simulink model "Taller4_TDCM"  (R2024a)
settings: Solver=VariableStepAuto  StartTime=0.0  StopTime=0.030  RelTol=1e-3
values from neighbouring files (symbols this model uses):
  A = [0 1; -1/(L*Cap) -R/L]    [Taller4_TCDM.m]    (also in Taller4_TCDM_v2.m)
  B = [0; 1/L]    [Taller4_TCDM.m]    (also in Taller4_TCDM_v2.m)
  C = [1/Cap 0]    [Taller4_TCDM.m]    (also in Taller4_TCDM_v2.m)
  D = 0    [Taller4_TCDM.m]    (also in Taller4_TCDM_v2.m)
  x0 = [0; 0]    [Taller4_TCDM_v2.m]
settings Model: Creator=emili  LastModifiedBy=emili

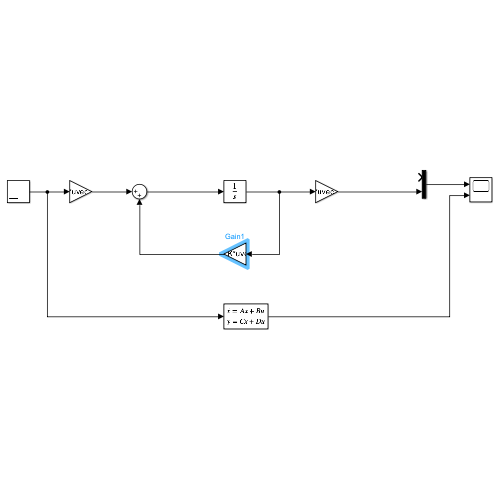
[thumbnail: Simulink's stored preview of the top-level diagram]
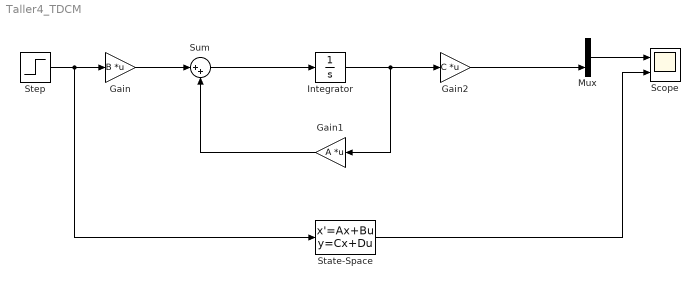
== system Taller4_TDCM ==
  Gain : Gain  Gain=B  Multiplication=Matrix(K*u) (u vector)
  Gain1 : Gain  Gain=A  Multiplication=Matrix(K*u) (u vector)
  Gain2 : Gain  Gain=C  Multiplication=Matrix(K*u) (u vector)
  Integrator : Integrator
  Mux : Mux  Inputs=2
  Scope : Scope  NumInputPorts=2
  State-Space : StateSpace  A=A  B=B  C=C  D=D  InitialCondition=x0
  Step : Step  Time=0.01  SampleTime=0.0001
  Sum : Sum  Inputs=|++
  wires:
  Mux/1 -> Scope/1
  Step/1 -> State-Space/1, Gain/1
  Gain/1 -> Sum/1
  Sum/1 -> Integrator/1
  Integrator/1 -> Gain1/1, Gain2/1
  Gain2/1 -> Mux/2
  Gain1/1 -> Sum/2
  State-Space/1 -> Scope/2
